simulink model "beamng_simulink_interface_demos_1"  (R2022b)
settings: Solver=FixedStepAuto  StartTime=0.0  StopTime=inf  FixedStep=0.0005  RelTol=1e-3
libraries: BeamNG_interface x1
settings Model: Creator=matti  LastModifiedBy=User
settings SolverCC: AlgebraicLoopSolver=TrustRegion
settings DebuggingCC: SFMachineParentedDataDiag=warning  ArithmeticOperatorsInVariantConditions=warning
settings SFSimCC: CustomCodeUndefinedFunction=UseInterfaceOnly

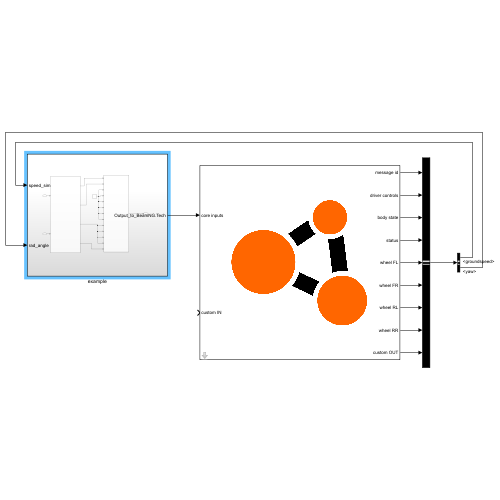
[thumbnail: Simulink's stored preview of the top-level diagram]
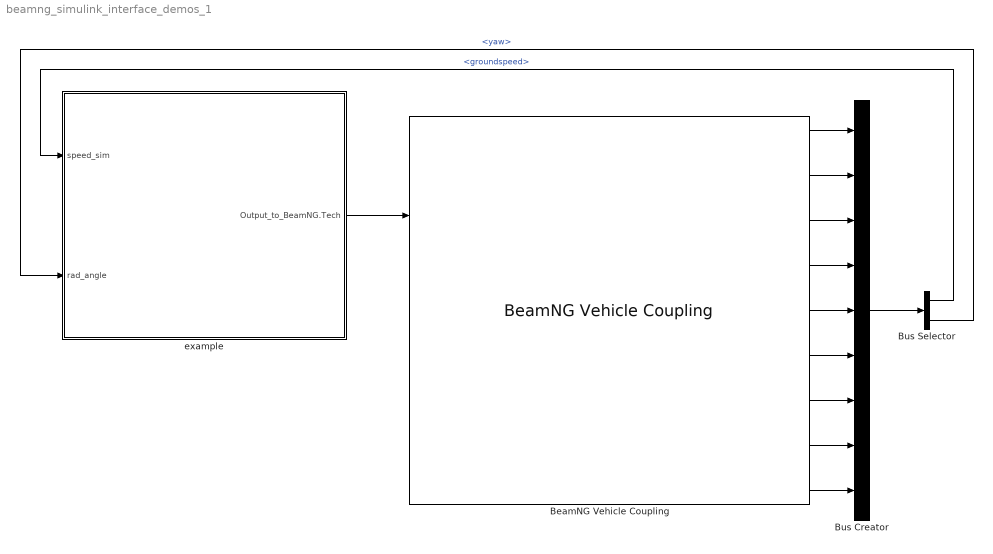
== system beamng_simulink_interface_demos_1 ==
  BeamNG Vehicle Coupling : BeamNG_interface/BeamNG Vehicle Coupling
      settings: SourceProductName=BeamNG
  Bus Creator : BusCreator  Inputs=9
  Bus Selector : BusSelector  OutputSignals=signal3.groundspeed,signal3.yaw
  example : Subsystem
  wires:
  Bus Creator/1 -> Bus Selector/1
  Bus Selector/1 -> example/1(speed_sim)  "<groundspeed>"
  Bus Selector/2 -> example/2(rad_angle)  "<yaw>"
  BeamNG Vehicle Coupling/1 -> Bus Creator/1
  BeamNG Vehicle Coupling/2 -> Bus Creator/2
  BeamNG Vehicle Coupling/3 -> Bus Creator/3
  BeamNG Vehicle Coupling/4 -> Bus Creator/4
  BeamNG Vehicle Coupling/5 -> Bus Creator/5
  BeamNG Vehicle Coupling/6 -> Bus Creator/6
  BeamNG Vehicle Coupling/7 -> Bus Creator/7
  BeamNG Vehicle Coupling/8 -> Bus Creator/8
  BeamNG Vehicle Coupling/9 -> Bus Creator/9
  example/1(Output_to_BeamNG.Tech) -> BeamNG Vehicle Coupling/1

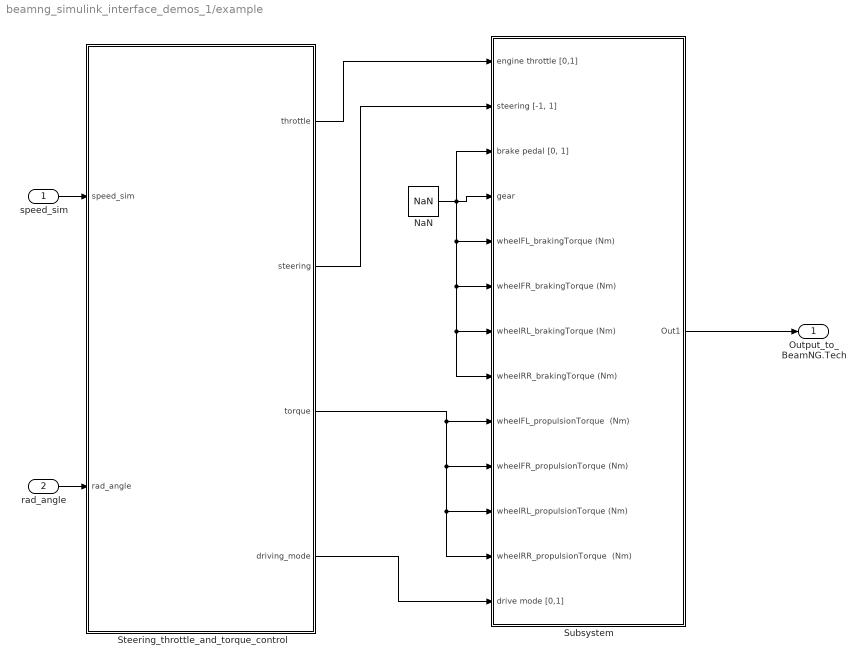
== system beamng_simulink_interface_demos_1/example ==
  speed_sim : Inport
  rad_angle : Inport  Port=2
  NaN : Constant  Value=NaN  OutDataTypeStr=Inherit: Inherit via back propagation
  Steering_throttle_and_torque_control : Subsystem
  Subsystem : Subsystem
  Output_to_BeamNG.Tech : Outport
  wires:
  rad_angle/1 -> Steering_throttle_and_torque_control/2(rad_angle)
  Subsystem/1(Out1) -> Output_to_BeamNG.Tech/1
  speed_sim/1 -> Steering_throttle_and_torque_control/1(speed_sim)
  Steering_throttle_and_torque_control/3(torque) -> Subsystem/10(wheelFR_propulsionTorque (Nm)), Subsystem/11(wheelRL_propulsionTorque (Nm)), Subsystem/12(wheelRR_propulsionTorque	 (Nm)), Subsystem/9(wheelFL_propulsionTorque	 (Nm))
  Steering_throttle_and_torque_control/4(driving_mode) -> Subsystem/13(drive mode [0,1])
  Steering_throttle_and_torque_control/2(steering) -> Subsystem/2("steering\t[-1, 1]")
  Steering_throttle_and_torque_control/1(throttle) -> Subsystem/1("engine throttle [0,1] ")
  NaN/1 -> Subsystem/3("brake pedal [0, 1]"), Subsystem/8("wheelRR_brakingTorque (Nm)\t"), Subsystem/7("wheelRL_brakingTorque (Nm)\t"), Subsystem/6("wheelFR_brakingTorque (Nm)\t"), Subsystem/5("wheelFL_brakingTorque (Nm)\t"), Subsystem/4("gear ")

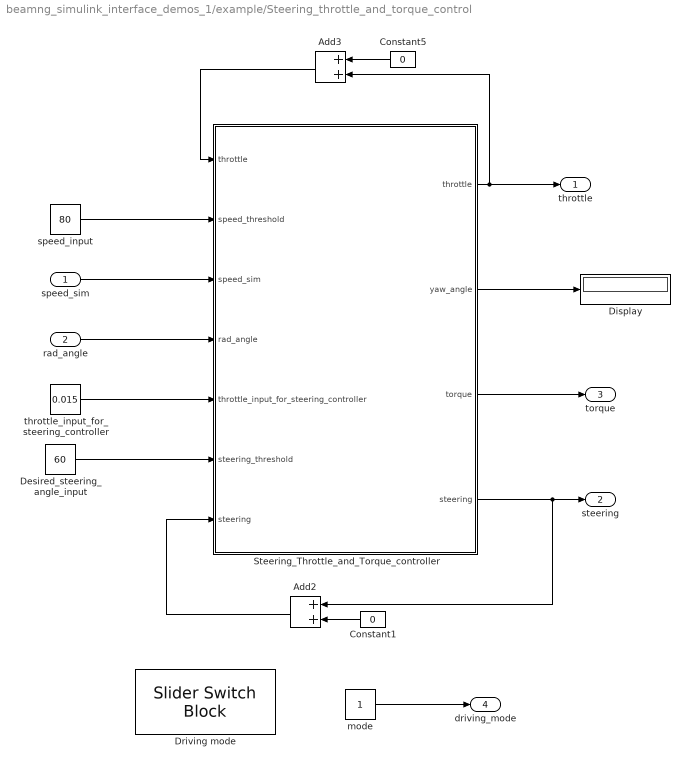
== system beamng_simulink_interface_demos_1/example/Steering_throttle_and_torque_control ==
  speed_sim : Inport
  rad_angle : Inport  Port=2
  Add2 : Sum
  Add3 : Sum
  Constant1 : Constant  Value=0
  Constant5 : Constant  Value=0
  Desired_steering_angle_input : Constant  Value=60
  Display : Display
  Driving mode : SliderSwitchBlock
      settings: Values={{'Torque', 'Pedal'}, [1 0]}
  Steering_Throttle_and_Torque_controller : MATLAB Function  TreatAsAtomicUnit=on
  mode : Constant
  speed_input : Constant  Value=80
  throttle_input_for_steering_controller : Constant  Value=0.015
  throttle : Outport
  steering : Outport  Port=2
  torque : Outport  Port=3
  driving_mode : Outport  Port=4
  wires:
  speed_input/1 -> Steering_Throttle_and_Torque_controller/2(speed_threshold)
  Desired_steering_angle_input/1 -> Steering_Throttle_and_Torque_controller/6(steering_threshold)
  Constant5/1 -> Add3/1
  Steering_Throttle_and_Torque_controller/1(throttle) -> Add3/2, throttle/1
  Add2/1 -> Steering_Throttle_and_Torque_controller/7("steering ")
  Constant1/1 -> Add2/2
  Add3/1 -> Steering_Throttle_and_Torque_controller/1("throttle ")
  mode/1 -> driving_mode/1
  Steering_Throttle_and_Torque_controller/3(torque) -> torque/1
  Steering_Throttle_and_Torque_controller/4(steering) -> Add2/1, steering/1
  rad_angle/1 -> Steering_Throttle_and_Torque_controller/4(rad_angle)
  speed_sim/1 -> Steering_Throttle_and_Torque_controller/3(speed_sim)
  throttle_input_for_steering_controller/1 -> Steering_Throttle_and_Torque_controller/5(throttle_input_for_steering_controller)
  Steering_Throttle_and_Torque_controller/2(yaw_angle) -> Display/1

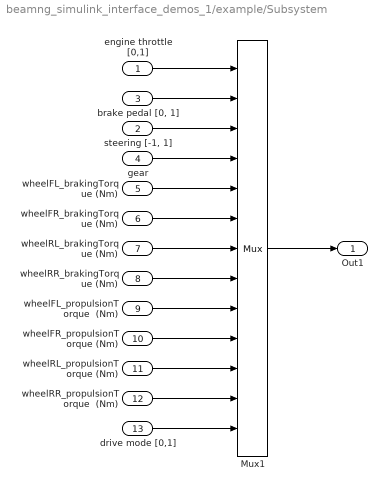
== system beamng_simulink_interface_demos_1/example/Subsystem ==
  "engine throttle [0,1] " : Inport
  "steering\t[-1, 1]" : Inport  Port=2
  "brake pedal [0, 1]" : Inport  Port=3
  "gear " : Inport  Port=4
  "wheelFL_brakingTorque (Nm)\t" : Inport  Port=5
  "wheelFR_brakingTorque (Nm)\t" : Inport  Port=6
  "wheelRL_brakingTorque (Nm)\t" : Inport  Port=7
  "wheelRR_brakingTorque (Nm)\t" : Inport  Port=8
  wheelFL_propulsionTorque	 (Nm) : Inport  Port=9
  wheelFR_propulsionTorque (Nm) : Inport  Port=10
  wheelRL_propulsionTorque (Nm) : Inport  Port=11
  wheelRR_propulsionTorque	 (Nm) : Inport  Port=12
  drive mode [0,1] : Inport  Port=13
  Mux1 : Mux  Inputs=13
  Out1 : Outport
  wires:
  "wheelFR_brakingTorque (Nm)\t"/1 -> Mux1/6
  "wheelRL_brakingTorque (Nm)\t"/1 -> Mux1/7
  "wheelRR_brakingTorque (Nm)\t"/1 -> Mux1/8
  "brake pedal [0, 1]"/1 -> Mux1/2
  drive mode [0,1]/1 -> Mux1/13
  wheelRR_propulsionTorque	 (Nm)/1 -> Mux1/12
  wheelFR_propulsionTorque (Nm)/1 -> Mux1/10
  wheelRL_propulsionTorque (Nm)/1 -> Mux1/11
  "wheelFL_brakingTorque (Nm)\t"/1 -> Mux1/5
  "engine throttle [0,1] "/1 -> Mux1/1
  "gear "/1 -> Mux1/4
  "steering\t[-1, 1]"/1 -> Mux1/3
  wheelFL_propulsionTorque	 (Nm)/1 -> Mux1/9
  Mux1/1 -> Out1/1

== matlab function beamng_simulink_interface_demos_1/example/Steering_throttle_and_torque_control/Steering_Throttle_and_Torque_controller ==
  data: throttle input; throttle output; yaw_angle output; torque output; steering output; speed_threshold input; speed_sim input; rad_angle input; throttle_input_for_steering_controller input; steering_threshold input; steering input
function [throttle,yaw_angle,torque,steering]= Controller(throttle,speed_threshold,speed_sim,rad_angle,throttle_input_for_steering_controller,steering_threshold,steering)
    % Steering 
    steering_clearance=1; % in degrees
    % here's converting the angle from radiant to degree      
    yaw_angle=rad_angle*(180/pi);
    if yaw_angle <= (steering_threshold-steering_clearance)
    steering=-throttle_input_for_steering_controller;
    end   

    if  yaw_angle > (steering_threshold)
    steering=throttle_input_for_steering_controller;
    end   


    % Throttle and Torque 
    speed_clearance=10;
    actual_speed=speed_sim*3.6;
    if actual_speed <= 5
    torque = 270 ; 
    throttle=0.5;
    elseif actual_speed <= (speed_threshold-speed_clearance)
    throttle=0.5;
    torque = 200 ; 
    elseif  actual_speed > (speed_threshold)
    throttle=-0.05;
    torque = 65; 
    else
    torque = 170; 
    end
    end
